simulink model "MIC_Mdl_Inverted_Pendulum"  (R2025b)
settings: Solver=ode15s  StartTime=0.0  StopTime=10  FixedStep=0.001  RelTol=1e-6  AbsTol=1e-6  EnableMultiTasking=on
values from neighbouring files (symbols this model uses):
  IdentTs = SimuRunInfo.IdentTs    [Compare.m]
  InitX = [0,0,6,0]    [Compare.m]
  ModelSelFlagLin = 4    [Compare.m]
  ModelSelFlagNonlin = ModelSelFlag    (= 3)    [Compare.m]
  TFPara = PhyPara    [Compare.m]
undefined symbols (not defined in the file or in its folder): NoisePara, UinDis, UinSin, UinSquare, WaveFlag
settings Model: Creator=wzj  LastModifiedBy=ASUS
settings SolverCC: AlgebraicLoopSolver=TrustRegion
settings DataIOCC: LimitDataPoints=on  SaveFormat=Array  ReturnWorkspaceOutputs=off
settings OptimizationCC: ReuseModelBlockBuffer=off  LifeSpan=inf
settings DebuggingCC: UnderspecifiedInitializationDetection=Classic  MergeDetectMultiDrivingBlocksExec=none  SolverPrmCheckMsg=warning  UnconnectedInputMsg=warning  UnconnectedOutputMsg=warning  UnconnectedLineMsg=warning  StateNameClashWarn=warning  SFUnexpectedBacktrackingDiag=warning  SFNoUnconditionalDefaultTransitionDiag=warning  SFExecutionAtInitializationDiag=none  ArithmeticOperatorsInVariantConditions=warning
settings HardwareCC: ProdBitPerPointer=32.0  ProdBitPerSizeT=32.0  ProdBitPerPtrDiffT=32.0  ProdLargestAtomicFloat=None  ProdIntDivRoundTo=Undefined  ProdEndianess=Unspecified  ProdWordSize=32.0  ProdHWDeviceType=32-bit Generic
settings ModelReferenceCC: EnableRefExpFcnMdlSchedulingChecks=on  PropagateSignalLabelsOutOfModel=off
settings SFSimCC: SimUseLocalCustomCode=off  CustomCodeUndefinedFunction=UseInterfaceOnly
settings RTWCC: RTWUseLocalCustomCode=off  GPUComputeCapability=3.5
settings CodeAppCC: StateflowObjectComments=on
settings GRTTargetCC: TargetLangStandard=C89/C90 (ANSI)
settings ConfigComp: CovMetricSettings=dw  CovSaveCumulativeToWorkspaceVar=on  CovSaveSingleToWorkspaceVar=on  CovExternalEMLEnable=off

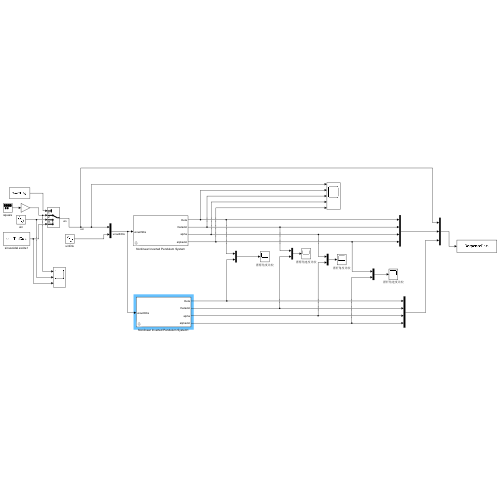
[thumbnail: Simulink's stored preview of the top-level diagram]
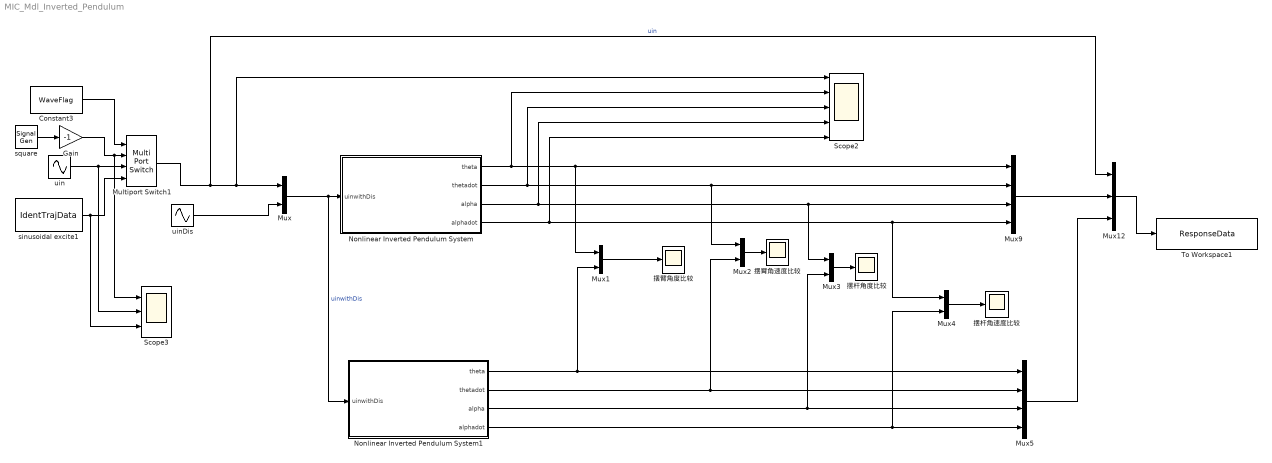
== system MIC_Mdl_Inverted_Pendulum ==
  Constant3 : Constant  Value=WaveFlag
  Gain : Gain  Gain=-1
  Multiport Switch1 : MultiPortSwitch  SaturateOnIntegerOverflow=off  InputSameDT=off
  Mux{,1..4} (5 alike) : Mux  Inputs=2
  Mux12 : Mux  Inputs=3
  Mux5 : Mux
  Mux9 : Mux
  Nonlinear Inverted Pendulum System : Subsystem  mask{TFPara=TFPara, ModelSelFlag=ModelSelFlagNonlin, InitX=InitX, NoisePara=NoisePara}
  Nonlinear Inverted Pendulum System1 : Subsystem  mask{TFPara=TFPara, ModelSelFlag=ModelSelFlagLin, InitX=InitX, NoisePara=NoisePara}
  Scope2 : Scope  NumInputPorts=5
      settings: ActiveDisplayYMinimum=-386.80995  ActiveDisplayYMaximum=3461.92632  DataLoggingSaveFormat=Structure
  Scope3 : Scope  NumInputPorts=3
      settings: ActiveDisplayYMinimum=0.09  ActiveDisplayYMaximum=0.11  DataLoggingVariableName=ScopeData2  DataLoggingSaveFormat=Structure
  To Workspace1 : ToWorkspace  VariableName=ResponseData  SaveFormat=Structure With Time  SampleTime=IdentTs
  sinusoidal excite1 : FromWorkspace  VariableName=IdentTrajData  SampleTime=IdentTs
  square : SignalGenerator  WaveForm=square  Amplitude=UinSquare(1)  Frequency=UinSquare(2)  Units=rad/sec
  uin : Sin  Amplitude=UinSin(1)  Bias=UinSin(3)  Frequency=UinSin(2)  SampleTime=0
  uinDis : Sin  Amplitude=UinDis(1)  Bias=UinDis(3)  Frequency=UinDis(2)  SampleTime=0
  摆杆角度比较 : Scope
      settings: ActiveDisplayYMinimum=-386.76037  ActiveDisplayYMaximum=3461.48007  DataLoggingVariableName=ScopeData10
  摆杆角速度比较 : Scope
      settings: ActiveDisplayYMinimum=-271.96904  ActiveDisplayYMaximum=271.97435  DataLoggingVariableName=ScopeData11
  摆臂角度比较 : Scope
      settings: ActiveDisplayYMinimum=-6.05868  ActiveDisplayYMaximum=6.37046  DataLoggingVariableName=ScopeData3
  摆臂角速度比较 : Scope
      settings: ActiveDisplayYMinimum=-56.65501  ActiveDisplayYMaximum=61.20032  DataLoggingVariableName=ScopeData9
  wires:
  Nonlinear Inverted Pendulum System1/4(alphadot) -> Mux5/4, Mux4/2
  Mux12/1 -> To Workspace1/1
  Mux9/1 -> Mux12/2
  Nonlinear Inverted Pendulum System/2(thetadot) -> Mux9/2, Mux2/1, Scope2/3
  Nonlinear Inverted Pendulum System1/3(alpha) -> Mux5/3, Mux3/2
  Nonlinear Inverted Pendulum System/1(theta) -> Mux9/1, Mux1/1, Scope2/2
  Mux4/1 -> 摆杆角速度比较/1
  Nonlinear Inverted Pendulum System/3(alpha) -> Mux9/3, Mux3/1, Scope2/4
  Nonlinear Inverted Pendulum System1/2(thetadot) -> Mux5/2, Mux2/2
  uinDis/1 -> Mux/2
  Constant3/1 -> Multiport Switch1/1
  sinusoidal excite1/1 -> Scope3/3, Multiport Switch1/4
  Nonlinear Inverted Pendulum System1/1(theta) -> Mux5/1, Mux1/2
  Multiport Switch1/1 -> Mux/1, Scope2/1, Mux12/1  "uin"
  uin/1 -> Scope3/2, Multiport Switch1/3
  Gain/1 -> Scope3/1, Multiport Switch1/2
  Mux/1 -> Nonlinear Inverted Pendulum System/1(uinwithDis), Nonlinear Inverted Pendulum System1/1(uinwithDis)  "uinwithDis"
  Mux2/1 -> 摆臂角速度比较/1
  square/1 -> Gain/1
  Nonlinear Inverted Pendulum System/4(alphadot) -> Mux9/4, Mux4/1, Scope2/5
  Mux1/1 -> 摆臂角度比较/1
  Mux3/1 -> 摆杆角度比较/1
  Mux5/1 -> Mux12/3

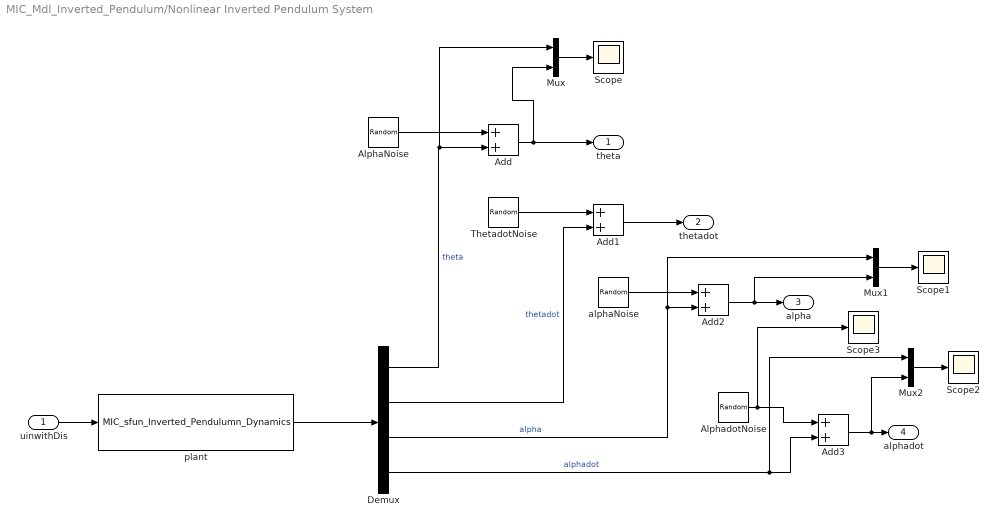
== system MIC_Mdl_Inverted_Pendulum/Nonlinear Inverted Pendulum System ==
  uinwithDis : Inport
  Add{,1..3} (4 alike) : Sum
  AlphaNoise : RandomNumber  Mean=NoisePara(1,1)  Variance=NoisePara(1,2)  Seed=NoisePara(1,3)  SampleTime=NoisePara(1,4)
  AlphadotNoise : RandomNumber  Mean=NoisePara(4,1)  Variance=NoisePara(4,2)  Seed=NoisePara(4,3)  SampleTime=NoisePara(4,4)
  Demux : Demux
  Mux : Mux  Inputs=2
  Mux1 : Mux  Inputs=2
  Mux2 : Mux  Inputs=2
  Scope{,1..3} (4 alike) : Scope
      Scope settings: ActiveDisplayYMinimum=-47.25618  ActiveDisplayYMaximum=49.39689
      Scope1 settings: ActiveDisplayYMinimum=-22.29261  ActiveDisplayYMaximum=130.5113  DataLoggingVariableName=ScopeData2
      Scope2 settings: ActiveDisplayYMinimum=-281.90197  ActiveDisplayYMaximum=281.82439  DataLoggingVariableName=ScopeData3
      Scope3 settings: ActiveDisplayYMinimum=-19.15922  ActiveDisplayYMaximum=20.14516  DataLoggingVariableName=ScopeData4
  ThetadotNoise : RandomNumber  Mean=NoisePara(2,1)  Variance=NoisePara(2,2)  Seed=NoisePara(2,3)  SampleTime=NoisePara(2,4)
  alphaNoise : RandomNumber  Mean=NoisePara(3,1)  Variance=NoisePara(3,2)  Seed=NoisePara(3,3)  SampleTime=NoisePara(3,4)
  plant : S-Function  FunctionName=MIC_sfun_Inverted_Pendulumn_Dynamics  Parameters=InitX,TFPara,ModelSelFlag  SFunctionDeploymentMode=off  EnableBusSupport=off
  theta : Outport
  thetadot : Outport  Port=2
  alpha : Outport  Port=3
  alphadot : Outport  Port=4
  wires:
  Demux/4 -> Mux2/1, Add3/2  "alphadot"
  Demux/3 -> Mux1/1, Add2/2  "alpha"
  uinwithDis/1 -> plant/1
  Demux/2 -> Add1/2  "thetadot"
  Demux/1 -> Mux/1, Add/2  "theta"
  AlphaNoise/1 -> Add/1
  Add/1 -> Mux/2, theta/1
  ThetadotNoise/1 -> Add1/1
  Add1/1 -> thetadot/1
  alphaNoise/1 -> Add2/1
  Add2/1 -> alpha/1, Mux1/2
  AlphadotNoise/1 -> Scope3/1, Add3/1
  Add3/1 -> Mux2/2, alphadot/1
  plant/1 -> Demux/1
  Mux/1 -> Scope/1
  Mux1/1 -> Scope1/1
  Mux2/1 -> Scope2/1

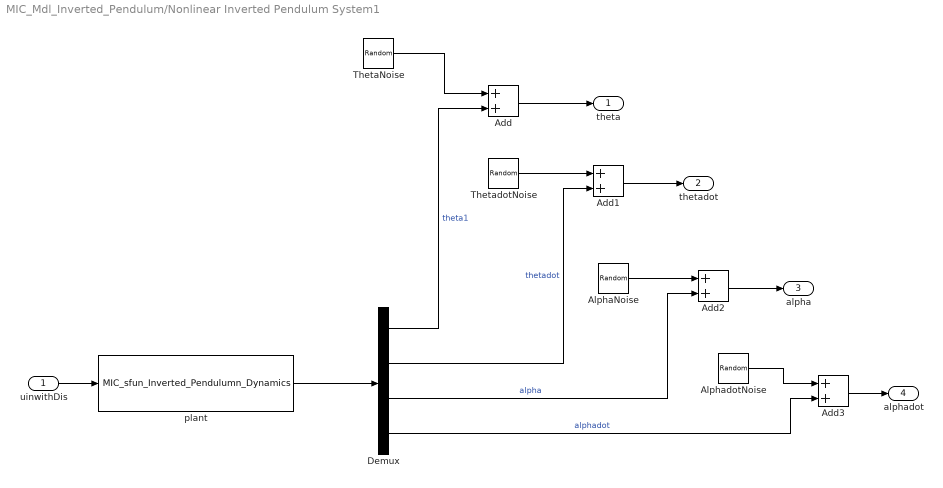
== system MIC_Mdl_Inverted_Pendulum/Nonlinear Inverted Pendulum System1 ==
  uinwithDis : Inport
  Add{,1..3} (4 alike) : Sum
  AlphaNoise : RandomNumber  Mean=NoisePara(3,1)  Variance=NoisePara(3,2)  Seed=NoisePara(3,3)  SampleTime=NoisePara(3,4)
  AlphadotNoise : RandomNumber  Mean=NoisePara(4,1)  Variance=NoisePara(4,2)  Seed=NoisePara(4,3)  SampleTime=NoisePara(4,4)
  Demux : Demux
  ThetaNoise : RandomNumber  Mean=NoisePara(1,1)  Variance=NoisePara(1,2)  Seed=NoisePara(1,3)  SampleTime=NoisePara(1,4)
  ThetadotNoise : RandomNumber  Mean=NoisePara(2,1)  Variance=NoisePara(2,2)  Seed=NoisePara(2,3)  SampleTime=NoisePara(2,4)
  plant : S-Function  FunctionName=MIC_sfun_Inverted_Pendulumn_Dynamics  Parameters=InitX,TFPara,ModelSelFlag  SFunctionDeploymentMode=off  EnableBusSupport=off
  theta : Outport
  thetadot : Outport  Port=2
  alpha : Outport  Port=3
  alphadot : Outport  Port=4
  wires:
  Demux/4 -> Add3/2  "alphadot"
  Demux/3 -> Add2/2  "alpha"
  uinwithDis/1 -> plant/1
  Demux/2 -> Add1/2  "thetadot"
  Demux/1 -> Add/2  "theta1"
  ThetaNoise/1 -> Add/1
  Add/1 -> theta/1
  ThetadotNoise/1 -> Add1/1
  Add1/1 -> thetadot/1
  AlphaNoise/1 -> Add2/1
  Add2/1 -> alpha/1
  AlphadotNoise/1 -> Add3/1
  Add3/1 -> alphadot/1
  plant/1 -> Demux/1
